simulink model "ARM_openloop_real"  (R2021a)
settings: Solver=VariableStepAuto  StartTime=0.0  StopTime=5  RelTol=1e-3  EnableMultiTasking=on
libraries: simulink x1, realtime_pacer_lib x1
settings Model: OrderedModelArguments=off  Creator=johnh  LastModifiedBy=Andy
settings SolverCC: AlgebraicLoopSolver=TrustRegion
settings DataIOCC: ReturnWorkspaceOutputs=off
settings OptimizationCC: LifeSpan=inf
settings DebuggingCC: SFUnexpectedBacktrackingDiag=warning  SFNoUnconditionalDefaultTransitionDiag=warning  SFExecutionAtInitializationDiag=none  SFMachineParentedDataDiag=warning  ArithmeticOperatorsInVariantConditions=warning
settings SFSimCC: SimUseLocalCustomCode=off  CustomCodeUndefinedFunction=UseInterfaceOnly
settings RTWCC: RTWUseLocalCustomCode=off
settings CodeAppCC: StateflowObjectComments=on
settings GRTTargetCC: TargetLangStandard=C89/C90 (ANSI)
settings ConfigComp: CovMetricSettings=dw  CovSaveCumulativeToWorkspaceVar=on  CovSaveSingleToWorkspaceVar=on  CovExternalEMLEnable=off

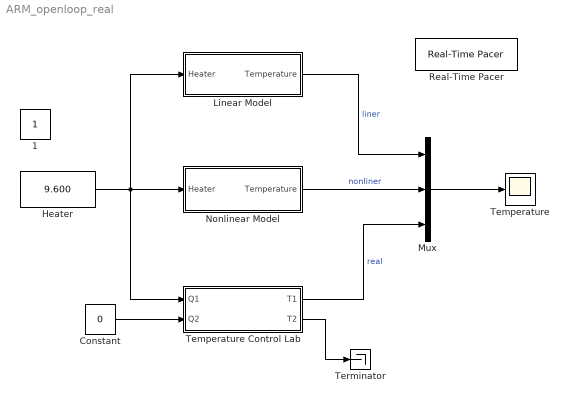
== system ARM_openloop_real ==
  Constant : Constant  Value=0
  Heater : simulink/Math Operations/Slider Gain  gain=9.600  low=0  high=120
  Linear Model : Subsystem
  Mux : Mux  Inputs=3
  Nonlinear Model : Subsystem
  Real-Time Pacer : realtime_pacer_lib/Real-Time Pacer  simTimePerRealTime=1
  Temperature : Scope
  Temperature Control Lab : Subsystem
  Terminator : Terminator
  1 : Constant  IOType=siggen
  wires:
  Mux/1 -> Temperature/1
  Linear Model/1(Temperature) -> Mux/1  "liner"
  Nonlinear Model/1(Temperature) -> Mux/2  "nonliner"
  Temperature Control Lab/1(T1) -> Mux/3  "real"
  Heater/1 -> Linear Model/1(Heater), Temperature Control Lab/1(Q1), Nonlinear Model/1(Heater)
  Constant/1 -> Temperature Control Lab/2(Q2)
  Temperature Control Lab/2(T2) -> Terminator/1

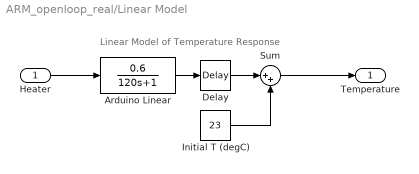
== system ARM_openloop_real/Linear Model ==
  note: Linear Model of Temperature Response
  Heater : Inport
  Arduino Linear : TransferFcn  Numerator=[0.6]  Denominator=[120 1]
  Delay : TransportDelay  DelayTime=3
  Initial T (degC) : Constant  Value=23
  Sum : Sum  Inputs=|++
  Temperature : Outport  VectorParamsAs1DForOutWhenUnconnected=off
  wires:
  Arduino Linear/1 -> Delay/1
  Delay/1 -> Sum/1
  Initial T (degC)/1 -> Sum/2
  Sum/1 -> Temperature/1
  Heater/1 -> Arduino Linear/1

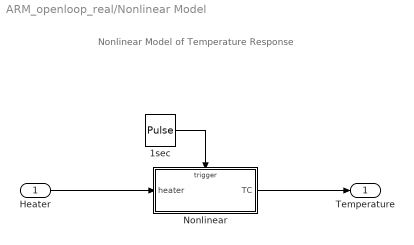
== system ARM_openloop_real/Nonlinear Model ==
  note: Nonlinear Model of Temperature Response
  Heater : Inport
  " Nonlinear" : Subsystem  TreatAsAtomicUnit=on
  1sec : DiscretePulseGenerator  PulseType=Time based  Period=1  PulseWidth=50
  Temperature : Outport  VectorParamsAs1DForOutWhenUnconnected=off
  wires:
  1sec/1 -> " Nonlinear"/Trigger
  " Nonlinear"/1(TC) -> Temperature/1
  Heater/1 -> " Nonlinear"/1(heater)

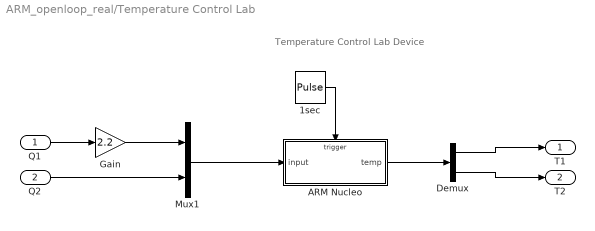
== system ARM_openloop_real/Temperature Control Lab ==
  note: Temperature Control Lab Device
  Q1 : Inport
  Q2 : Inport  Port=2
  1sec : DiscretePulseGenerator  PulseType=Time based  Period=1  PulseWidth=50
  ARM Nucleo : Subsystem  TreatAsAtomicUnit=on
  Demux : Demux  Outputs=2
  Gain : Gain  Gain=2.2
  Mux1 : Mux  Inputs=2
  T1 : Outport  VectorParamsAs1DForOutWhenUnconnected=off
  T2 : Outport  Port=2  VectorParamsAs1DForOutWhenUnconnected=off
  wires:
  1sec/1 -> ARM Nucleo/Trigger
  Mux1/1 -> ARM Nucleo/1(input)
  Q1/1 -> Gain/1
  Q2/1 -> Mux1/2
  Gain/1 -> Mux1/1
  ARM Nucleo/1(temp) -> Demux/1
  Demux/1 -> T1/1
  Demux/2 -> T2/1

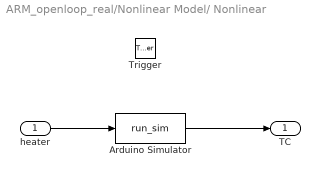
== system ARM_openloop_real/Nonlinear Model/ Nonlinear ==
  heater : Inport
  Trigger : TriggerPort  VariantControl=Variant
  Arduino Simulator : MATLABFcn  MATLABFcn=run_sim
  TC : Outport  InitialOutput=23  VectorParamsAs1DForOutWhenUnconnected=off
  wires:
  heater/1 -> Arduino Simulator/1
  Arduino Simulator/1 -> TC/1

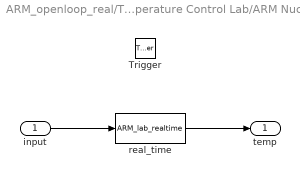
== system ARM_openloop_real/Temperature Control Lab/ARM Nucleo ==
  input : Inport  LatchByDelayingOutsideSignal=on
  Trigger : TriggerPort  VariantControl=Variant
  real_time : MATLABFcn  MATLABFcn=ARM_lab_realtime  Output1D=off
  temp : Outport  InitialOutput=25  VectorParamsAs1DForOutWhenUnconnected=off
  wires:
  input/1 -> real_time/1
  real_time/1 -> temp/1
